simulink library "Word_Multiplexers_Lib"  (Simulink 8.7)
settings: Solver=ode45  StartTime=0.0  StopTime=10.0  RelTol=1e-3
(part 2 of 3)

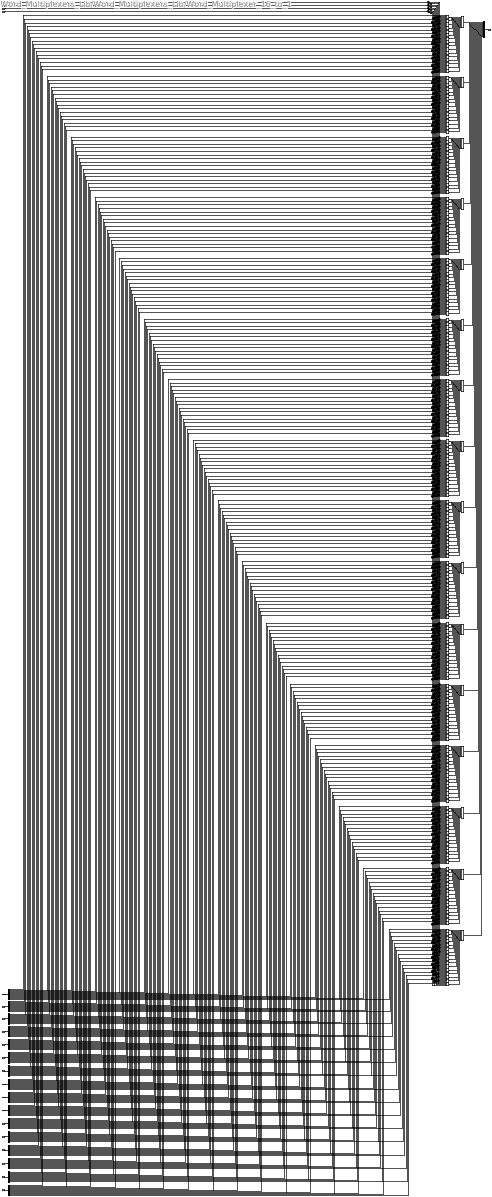
== system Word_Multiplexers_Lib/Word_Multiplexers_Lib/Word_Multiplexer_16_to_1 ==
  note: Bit_Multiplexer_16_to_1(Bit_15)
  note: Bit_Multiplexer_16_to_1(Bit_14)
  note: Bit_Multiplexer_16_to_1(Bit_13)
  note: Bit_Multiplexer_16_to_1(Bit_12)
  note: Bit_Multiplexer_16_to_1(Bit_11)
  note: Bit_Multiplexer_16_to_1(Bit_10)
  note: Bit_Multiplexer_16_to_1(Bit_09)
  note: Bit_Multiplexer_16_to_1(Bit_08)
  note: Bit_Multiplexer_16_to_1(Bit_07)
  note: Bit_Multiplexer_16_to_1(Bit_06)
  note: Bit_Multiplexer_16_to_1(Bit_05)
  note: Bit_Multiplexer_16_to_1(Bit_04)
  note: Bit_Multiplexer_16_to_1(Bit_03)
  note: Bit_Multiplexer_16_to_1(Bit_02)
  note: Bit_Multiplexer_16_to_1(Bit_01)
  note: Bit_Multiplexer_16_to_1(Bit_00)
  Address_3(1b) : Inport
  Address_2(1b) : Inport  Port=2
  Address_1(1b) : Inport  Port=3
  Address_0(1b) : Inport  Port=4
  Data_In_15(2B) : Inport  Port=5
  Data_In_14(2B) : Inport  Port=6
  Data_In_13(2B) : Inport  Port=7
  Data_In_12(2B) : Inport  Port=8
  Data_In_11(2B) : Inport  Port=9
  Data_In_10(2B) : Inport  Port=10
  Data_In_09(2B) : Inport  Port=11
  Data_In_08(2B) : Inport  Port=12
  Data_In_07(2B) : Inport  Port=13
  Data_In_06(2B) : Inport  Port=14
  Data_In_05(2B) : Inport  Port=15
  Data_In_04(2B) : Inport  Port=16
  Data_In_03(2B) : Inport  Port=17
  Data_In_02(2B) : Inport  Port=18
  Data_In_01(2B) : Inport  Port=19
  Data_In_00(2B) : Inport  Port=20
  Bus Creator : BusCreator  Inputs=16
  Bus Selector{,1..15} (16 alike) : BusSelector  OutputSignals=signal1,signal2,signal3,signal4,signal5,signal6,signal7,signal8,signal9,signal10,signal11,signal12,signal13,signal14,signal15,signal16
  Logical Operator{,1..7,13..22,26..39,42..43,47..60,63..64,68..81,84..85,89..102,105..106,110..123,126..127,131..144,147..148,152..165,168..169,173..186,189..190,194..207,210..211,215..228,231..232,236..249,252..253,257..270,273..274,278..291,294..295,299..312,315..316,320..333} (256 alike) : Logic  Inputs=5  IconShape=distinctive  AllPortsSameDT=off  OutDataTypeStr=boolean
  Logical Operator{8,40,61,82,103,124,145,166,187,208,229,250,271,292,313,334} (16 alike) : Logic  Operator=OR  Inputs=16  IconShape=distinctive  OutDataTypeStr=boolean
  Logical Operator{317..319,335} (4 alike) : Logic  Operator=NOT  Inputs=4  IconShape=distinctive  AllPortsSameDT=off  OutDataTypeStr=boolean
  Data_Out(2B) : Outport
  wires:
  Data_In_15(2B)/1 -> Bus Selector15/1
  Logical Operator103/1 -> Bus Creator/12
  Logical Operator124/1 -> Bus Creator/11
  Logical Operator145/1 -> Bus Creator/10
  Logical Operator166/1 -> Bus Creator/9
  Logical Operator82/1 -> Bus Creator/13
  Logical Operator61/1 -> Bus Creator/14
  Logical Operator40/1 -> Bus Creator/15
  Logical Operator8/1 -> Bus Creator/16
  Data_In_14(2B)/1 -> Bus Selector14/1
  Data_In_13(2B)/1 -> Bus Selector13/1
  Data_In_12(2B)/1 -> Bus Selector12/1
  Data_In_11(2B)/1 -> Bus Selector11/1
  Data_In_10(2B)/1 -> Bus Selector10/1
  Data_In_09(2B)/1 -> Bus Selector9/1
  Data_In_08(2B)/1 -> Bus Selector8/1
  Data_In_07(2B)/1 -> Bus Selector7/1
  Data_In_06(2B)/1 -> Bus Selector6/1
  Data_In_05(2B)/1 -> Bus Selector5/1
  Data_In_04(2B)/1 -> Bus Selector4/1
  Data_In_03(2B)/1 -> Bus Selector3/1
  Data_In_02(2B)/1 -> Bus Selector2/1
  Data_In_01(2B)/1 -> Bus Selector1/1
  Data_In_00(2B)/1 -> Bus Selector/1
  Bus Creator/1 -> Data_Out(2B)/1
  Logical Operator271/1 -> Bus Creator/4
  Logical Operator292/1 -> Bus Creator/3
  Logical Operator313/1 -> Bus Creator/2
  Logical Operator334/1 -> Bus Creator/1
  Logical Operator250/1 -> Bus Creator/5
  Logical Operator229/1 -> Bus Creator/6
  Logical Operator208/1 -> Bus Creator/7
  Logical Operator187/1 -> Bus Creator/8
  Logical Operator319/1 -> Logical Operator316/5, Logical Operator329/5, Logical Operator331/5, Logical Operator333/5, Logical Operator321/5, Logical Operator323/5, Logical Operator325/5, Logical Operator1/5, Logical Operator3/5, Logical Operator5/5, Logical Operator7/5, Logical Operator14/5, Logical Operator16/5, Logical Operator18/5, Logical Operator20/5, Logical Operator34/5, Logical Operator31/5, Logical Operator29/5, Logical Operator27/5, Logical Operator39/5, Logical Operator37/5, Logical Operator35/5, Logical Operator22/5, Logical Operator55/5, Logical Operator52/5, Logical Operator50/5, Logical Operator48/5, Logical Operator60/5, Logical Operator58/5, Logical Operator56/5, Logical Operator43/5, Logical Operator76/5, Logical Operator73/5, Logical Operator71/5, Logical Operator69/5, Logical Operator81/5, Logical Operator79/5, Logical Operator77/5, Logical Operator64/5, Logical Operator97/5, Logical Operator94/5, Logical Operator92/5, Logical Operator90/5, Logical Operator102/5, Logical Operator100/5, Logical Operator98/5, Logical Operator85/5, Logical Operator118/5, Logical Operator115/5, Logical Operator113/5, Logical Operator111/5, Logical Operator123/5, Logical Operator121/5, Logical Operator119/5, Logical Operator106/5, Logical Operator139/5, Logical Operator136/5, Logical Operator134/5, Logical Operator132/5, Logical Operator144/5, Logical Operator142/5, Logical Operator140/5, Logical Operator127/5, Logical Operator160/5, Logical Operator157/5, Logical Operator155/5, Logical Operator153/5, Logical Operator165/5, Logical Operator163/5, Logical Operator161/5, Logical Operator148/5, Logical Operator181/5, Logical Operator178/5, Logical Operator176/5, Logical Operator174/5, Logical Operator186/5, Logical Operator184/5, Logical Operator182/5, Logical Operator169/5, Logical Operator202/5, Logical Operator199/5, Logical Operator197/5, Logical Operator195/5, Logical Operator207/5, Logical Operator205/5, Logical Operator203/5, Logical Operator190/5, Logical Operator223/5, Logical Operator220/5, Logical Operator218/5, Logical Operator216/5, Logical Operator228/5, Logical Operator226/5, Logical Operator224/5, Logical Operator211/5, Logical Operator244/5, Logical Operator241/5, Logical Operator239/5, Logical Operator237/5, Logical Operator249/5, Logical Operator247/5, Logical Operator245/5, Logical Operator232/5, Logical Operator265/5, Logical Operator262/5, Logical Operator260/5, Logical Operator258/5, Logical Operator270/5, Logical Operator268/5, Logical Operator266/5, Logical Operator253/5, Logical Operator286/5, Logical Operator283/5, Logical Operator281/5, Logical Operator279/5, Logical Operator291/5, Logical Operator289/5, Logical Operator287/5, Logical Operator274/5, Logical Operator307/5, Logical Operator304/5, Logical Operator302/5, Logical Operator300/5, Logical Operator312/5, Logical Operator310/5, Logical Operator308/5, Logical Operator295/5, Logical Operator328/5
  Logical Operator318/1 -> Logical Operator327/4, Logical Operator329/4, Logical Operator332/4, Logical Operator333/4, Logical Operator322/4, Logical Operator323/4, Logical Operator326/4, Logical Operator34/4, Logical Operator2/4, Logical Operator3/4, Logical Operator6/4, Logical Operator7/4, Logical Operator15/4, Logical Operator16/4, Logical Operator19/4, Logical Operator20/4, Logical Operator32/4, Logical Operator29/4, Logical Operator28/4, Logical Operator39/4, Logical Operator38/4, Logical Operator35/4, Logical Operator33/4, Logical Operator55/4, Logical Operator53/4, Logical Operator50/4, Logical Operator49/4, Logical Operator60/4, Logical Operator59/4, Logical Operator56/4, Logical Operator54/4, Logical Operator76/4, Logical Operator74/4, Logical Operator71/4, Logical Operator70/4, Logical Operator81/4, Logical Operator80/4, Logical Operator77/4, Logical Operator75/4, Logical Operator97/4, Logical Operator95/4, Logical Operator92/4, Logical Operator91/4, Logical Operator102/4, Logical Operator101/4, Logical Operator98/4, Logical Operator96/4, Logical Operator118/4, Logical Operator116/4, Logical Operator113/4, Logical Operator112/4, Logical Operator123/4, Logical Operator122/4, Logical Operator119/4, Logical Operator117/4, Logical Operator139/4, Logical Operator137/4, Logical Operator134/4, Logical Operator133/4, Logical Operator144/4, Logical Operator143/4, Logical Operator140/4, Logical Operator138/4, Logical Operator160/4, Logical Operator158/4, Logical Operator155/4, Logical Operator154/4, Logical Operator165/4, Logical Operator164/4, Logical Operator161/4, Logical Operator159/4, Logical Operator181/4, Logical Operator179/4, Logical Operator176/4, Logical Operator175/4, Logical Operator186/4, Logical Operator185/4, Logical Operator182/4, Logical Operator180/4, Logical Operator202/4, Logical Operator200/4, Logical Operator197/4, Logical Operator196/4, Logical Operator207/4, Logical Operator206/4, Logical Operator203/4, Logical Operator201/4, Logical Operator223/4, Logical Operator221/4, Logical Operator218/4, Logical Operator217/4, Logical Operator228/4, Logical Operator227/4, Logical Operator224/4, Logical Operator222/4, Logical Operator244/4, Logical Operator242/4, Logical Operator239/4, Logical Operator238/4, Logical Operator249/4, Logical Operator248/4, Logical Operator245/4, Logical Operator243/4, Logical Operator265/4, Logical Operator263/4, Logical Operator260/4, Logical Operator259/4, Logical Operator270/4, Logical Operator269/4, Logical Operator266/4, Logical Operator264/4, Logical Operator286/4, Logical Operator284/4, Logical Operator281/4, Logical Operator280/4, Logical Operator291/4, Logical Operator290/4, Logical Operator287/4, Logical Operator285/4, Logical Operator307/4, Logical Operator305/4, Logical Operator302/4, Logical Operator301/4, Logical Operator312/4, Logical Operator311/4, Logical Operator308/4, Logical Operator306/4, Logical Operator328/4
  Logical Operator317/1 -> Logical Operator330/3, Logical Operator331/3, Logical Operator332/3, Logical Operator333/3, Logical Operator324/3, Logical Operator325/3, Logical Operator326/3, Logical Operator34/3, Logical Operator4/3, Logical Operator5/3, Logical Operator6/3, Logical Operator7/3, Logical Operator17/3, Logical Operator18/3, Logical Operator19/3, Logical Operator20/3, Logical Operator32/3, Logical Operator31/3, Logical Operator30/3, Logical Operator39/3, Logical Operator38/3, Logical Operator37/3, Logical Operator36/3, Logical Operator55/3, Logical Operator53/3, Logical Operator52/3, Logical Operator51/3, Logical Operator60/3, Logical Operator59/3, Logical Operator58/3, Logical Operator57/3, Logical Operator76/3, Logical Operator74/3, Logical Operator73/3, Logical Operator72/3, Logical Operator81/3, Logical Operator80/3, Logical Operator79/3, Logical Operator78/3, Logical Operator97/3, Logical Operator95/3, Logical Operator94/3, Logical Operator93/3, Logical Operator102/3, Logical Operator101/3, Logical Operator100/3, Logical Operator99/3, Logical Operator118/3, Logical Operator116/3, Logical Operator115/3, Logical Operator114/3, Logical Operator123/3, Logical Operator122/3, Logical Operator121/3, Logical Operator120/3, Logical Operator139/3, Logical Operator137/3, Logical Operator136/3, Logical Operator135/3, Logical Operator144/3, Logical Operator143/3, Logical Operator142/3, Logical Operator141/3, Logical Operator160/3, Logical Operator158/3, Logical Operator157/3, Logical Operator156/3, Logical Operator165/3, Logical Operator164/3, Logical Operator163/3, Logical Operator162/3, Logical Operator181/3, Logical Operator179/3, Logical Operator178/3, Logical Operator177/3, Logical Operator186/3, Logical Operator185/3, Logical Operator184/3, Logical Operator183/3, Logical Operator202/3, Logical Operator200/3, Logical Operator199/3, Logical Operator198/3, Logical Operator207/3, Logical Operator206/3, Logical Operator205/3, Logical Operator204/3, Logical Operator223/3, Logical Operator221/3, Logical Operator220/3, Logical Operator219/3, Logical Operator228/3, Logical Operator227/3, Logical Operator226/3, Logical Operator225/3, Logical Operator244/3, Logical Operator242/3, Logical Operator241/3, Logical Operator240/3, Logical Operator249/3, Logical Operator248/3, Logical Operator247/3, Logical Operator246/3, Logical Operator265/3, Logical Operator263/3, Logical Operator262/3, Logical Operator261/3, Logical Operator270/3, Logical Operator269/3, Logical Operator268/3, Logical Operator267/3, Logical Operator286/3, Logical Operator284/3, Logical Operator283/3, Logical Operator282/3, Logical Operator291/3, Logical Operator290/3, Logical Operator289/3, Logical Operator288/3, Logical Operator307/3, Logical Operator305/3, Logical Operator304/3, Logical Operator303/3, Logical Operator312/3, Logical Operator311/3, Logical Operator310/3, Logical Operator309/3, Logical Operator328/3
  Logical Operator335/1 -> Logical Operator320/2, Logical Operator321/2, Logical Operator322/2, Logical Operator323/2, Logical Operator324/2, Logical Operator325/2, Logical Operator326/2, Logical Operator34/2, Logical Operator13/2, Logical Operator14/2, Logical Operator15/2, Logical Operator16/2, Logical Operator17/2, Logical Operator18/2, Logical Operator19/2, Logical Operator20/2, Logical Operator32/2, Logical Operator31/2, Logical Operator30/2, Logical Operator29/2, Logical Operator28/2, Logical Operator27/2, Logical Operator26/2, Logical Operator55/2, Logical Operator53/2, Logical Operator52/2, Logical Operator51/2, Logical Operator50/2, Logical Operator49/2, Logical Operator48/2, Logical Operator47/2, Logical Operator76/2, Logical Operator74/2, Logical Operator73/2, Logical Operator72/2, Logical Operator71/2, Logical Operator70/2, Logical Operator69/2, Logical Operator68/2, Logical Operator97/2, Logical Operator95/2, Logical Operator94/2, Logical Operator93/2, Logical Operator92/2, Logical Operator91/2, Logical Operator90/2, Logical Operator89/2, Logical Operator118/2, Logical Operator116/2, Logical Operator115/2, Logical Operator114/2, Logical Operator113/2, Logical Operator112/2, Logical Operator111/2, Logical Operator110/2, Logical Operator139/2, Logical Operator137/2, Logical Operator136/2, Logical Operator135/2, Logical Operator134/2, Logical Operator133/2, Logical Operator132/2, Logical Operator131/2, Logical Operator160/2, Logical Operator158/2, Logical Operator157/2, Logical Operator156/2, Logical Operator155/2, Logical Operator154/2, Logical Operator153/2, Logical Operator152/2, Logical Operator181/2, Logical Operator179/2, Logical Operator178/2, Logical Operator177/2, Logical Operator176/2, Logical Operator175/2, Logical Operator174/2, Logical Operator173/2, Logical Operator202/2, Logical Operator200/2, Logical Operator199/2, Logical Operator198/2, Logical Operator197/2, Logical Operator196/2, Logical Operator195/2, Logical Operator194/2, Logical Operator223/2, Logical Operator221/2, Logical Operator220/2, Logical Operator219/2, Logical Operator218/2, Logical Operator217/2, Logical Operator216/2, Logical Operator215/2, Logical Operator244/2, Logical Operator242/2, Logical Operator241/2, Logical Operator240/2, Logical Operator239/2, Logical Operator238/2, Logical Operator237/2, Logical Operator236/2, Logical Operator265/2, Logical Operator263/2, Logical Operator262/2, Logical Operator261/2, Logical Operator260/2, Logical Operator259/2, Logical Operator258/2, Logical Operator257/2, Logical Operator286/2, Logical Operator284/2, Logical Operator283/2, Logical Operator282/2, Logical Operator281/2, Logical Operator280/2, Logical Operator279/2, Logical Operator278/2, Logical Operator307/2, Logical Operator305/2, Logical Operator304/2, Logical Operator303/2, Logical Operator302/2, Logical Operator301/2, Logical Operator300/2, Logical Operator299/2, Logical Operator328/2
  Bus Selector/16 -> Logical Operator20/1  "<signal16>"
  Bus Selector1/16 -> Logical Operator19/1  "<signal16>"
  Bus Selector2/16 -> Logical Operator18/1  "<signal16>"
  Bus Selector3/16 -> Logical Operator17/1  "<signal16>"
  Bus Selector4/16 -> Logical Operator16/1  "<signal16>"
  Bus Selector5/16 -> Logical Operator15/1  "<signal16>"
  Bus Selector6/16 -> Logical Operator14/1  "<signal16>"
  Bus Selector7/16 -> Logical Operator13/1  "<signal16>"
  Logical Operator20/1 -> Logical Operator8/16
  Logical Operator19/1 -> Logical Operator8/15
  Logical Operator18/1 -> Logical Operator8/14
  Logical Operator17/1 -> Logical Operator8/13
  Logical Operator16/1 -> Logical Operator8/12
  Logical Operator15/1 -> Logical Operator8/11
  Logical Operator14/1 -> Logical Operator8/10
  Logical Operator13/1 -> Logical Operator8/9
  Bus Selector15/16 -> Logical Operator/1  "<signal16>"
  Bus Selector14/16 -> Logical Operator1/1  "<signal16>"
  Bus Selector13/16 -> Logical Operator2/1  "<signal16>"
  Bus Selector12/16 -> Logical Operator3/1  "<signal16>"
  Bus Selector11/16 -> Logical Operator4/1  "<signal16>"
  Bus Selector10/16 -> Logical Operator5/1  "<signal16>"
  Bus Selector9/16 -> Logical Operator6/1  "<signal16>"
  Bus Selector8/16 -> Logical Operator7/1  "<signal16>"
  Logical Operator7/1 -> Logical Operator8/8
  Logical Operator6/1 -> Logical Operator8/7
  Logical Operator5/1 -> Logical Operator8/6
  Logical Operator4/1 -> Logical Operator8/5
  Logical Operator3/1 -> Logical Operator8/4
  Logical Operator2/1 -> Logical Operator8/3
  Logical Operator1/1 -> Logical Operator8/2
  Logical Operator/1 -> Logical Operator8/1
  Bus Selector/15 -> Logical Operator34/1  "<signal15>"
  Bus Selector1/15 -> Logical Operator32/1  "<signal15>"
  Bus Selector2/15 -> Logical Operator31/1  "<signal15>"
  Bus Selector3/15 -> Logical Operator30/1  "<signal15>"
  Bus Selector4/15 -> Logical Operator29/1  "<signal15>"
  Bus Selector5/15 -> Logical Operator28/1  "<signal15>"
  Bus Selector6/15 -> Logical Operator27/1  "<signal15>"
  Bus Selector7/15 -> Logical Operator26/1  "<signal15>"
  Logical Operator34/1 -> Logical Operator40/16
  Logical Operator32/1 -> Logical Operator40/15
  Logical Operator31/1 -> Logical Operator40/14
  Logical Operator30/1 -> Logical Operator40/13
  Logical Operator29/1 -> Logical Operator40/12
  Logical Operator28/1 -> Logical Operator40/11
  Logical Operator27/1 -> Logical Operator40/10
  Logical Operator26/1 -> Logical Operator40/9
  Bus Selector15/15 -> Logical Operator21/1  "<signal15>"
  Bus Selector14/15 -> Logical Operator22/1  "<signal15>"
  Bus Selector13/15 -> Logical Operator33/1  "<signal15>"
  Bus Selector12/15 -> Logical Operator35/1  "<signal15>"
  Bus Selector11/15 -> Logical Operator36/1  "<signal15>"
  Bus Selector10/15 -> Logical Operator37/1  "<signal15>"
  Bus Selector9/15 -> Logical Operator38/1  "<signal15>"
  Bus Selector8/15 -> Logical Operator39/1  "<signal15>"
  Logical Operator39/1 -> Logical Operator40/8
  Logical Operator38/1 -> Logical Operator40/7
  Logical Operator37/1 -> Logical Operator40/6
  Logical Operator36/1 -> Logical Operator40/5
  Logical Operator35/1 -> Logical Operator40/4
  Logical Operator33/1 -> Logical Operator40/3
  Logical Operator22/1 -> Logical Operator40/2
  Logical Operator21/1 -> Logical Operator40/1
  Bus Selector/14 -> Logical Operator55/1  "<signal14>"
  Bus Selector1/14 -> Logical Operator53/1  "<signal14>"
  Bus Selector2/14 -> Logical Operator52/1  "<signal14>"
  Bus Selector3/14 -> Logical Operator51/1  "<signal14>"
  Bus Selector4/14 -> Logical Operator50/1  "<signal14>"
  Bus Selector5/14 -> Logical Operator49/1  "<signal14>"
  Bus Selector6/14 -> Logical Operator48/1  "<signal14>"
  Bus Selector7/14 -> Logical Operator47/1  "<signal14>"
  Logical Operator55/1 -> Logical Operator61/16
  Logical Operator53/1 -> Logical Operator61/15
  Logical Operator52/1 -> Logical Operator61/14
  Logical Operator51/1 -> Logical Operator61/13
  Logical Operator50/1 -> Logical Operator61/12
  Logical Operator49/1 -> Logical Operator61/11
  Logical Operator48/1 -> Logical Operator61/10
  Logical Operator47/1 -> Logical Operator61/9
  Bus Selector15/14 -> Logical Operator42/1  "<signal14>"
  Bus Selector14/14 -> Logical Operator43/1  "<signal14>"
  Bus Selector13/14 -> Logical Operator54/1  "<signal14>"
  Bus Selector12/14 -> Logical Operator56/1  "<signal14>"
  Bus Selector11/14 -> Logical Operator57/1  "<signal14>"
  Bus Selector10/14 -> Logical Operator58/1  "<signal14>"
  Bus Selector9/14 -> Logical Operator59/1  "<signal14>"
  Bus Selector8/14 -> Logical Operator60/1  "<signal14>"
  Logical Operator60/1 -> Logical Operator61/8
  Logical Operator59/1 -> Logical Operator61/7
  Logical Operator58/1 -> Logical Operator61/6
  Logical Operator57/1 -> Logical Operator61/5
  Logical Operator56/1 -> Logical Operator61/4
  Logical Operator54/1 -> Logical Operator61/3
  Logical Operator43/1 -> Logical Operator61/2
  Logical Operator42/1 -> Logical Operator61/1
  Bus Selector/13 -> Logical Operator76/1  "<signal13>"
  Bus Selector1/13 -> Logical Operator74/1  "<signal13>"
  Bus Selector2/13 -> Logical Operator73/1  "<signal13>"
  Bus Selector3/13 -> Logical Operator72/1  "<signal13>"
  Bus Selector4/13 -> Logical Operator71/1  "<signal13>"
  Bus Selector5/13 -> Logical Operator70/1  "<signal13>"
  Bus Selector6/13 -> Logical Operator69/1  "<signal13>"
  Bus Selector7/13 -> Logical Operator68/1  "<signal13>"
  Logical Operator76/1 -> Logical Operator82/16
  Logical Operator74/1 -> Logical Operator82/15
  Logical Operator73/1 -> Logical Operator82/14
  Logical Operator72/1 -> Logical Operator82/13
  Logical Operator71/1 -> Logical Operator82/12
  Logical Operator70/1 -> Logical Operator82/11
  Logical Operator69/1 -> Logical Operator82/10
  Logical Operator68/1 -> Logical Operator82/9
  Bus Selector15/13 -> Logical Operator63/1  "<signal13>"
  Bus Selector14/13 -> Logical Operator64/1  "<signal13>"
  Bus Selector13/13 -> Logical Operator75/1  "<signal13>"
  Bus Selector12/13 -> Logical Operator77/1  "<signal13>"
  Bus Selector11/13 -> Logical Operator78/1  "<signal13>"
  Bus Selector10/13 -> Logical Operator79/1  "<signal13>"
  Bus Selector9/13 -> Logical Operator80/1  "<signal13>"
  Bus Selector8/13 -> Logical Operator81/1  "<signal13>"
  Logical Operator81/1 -> Logical Operator82/8
  Logical Operator80/1 -> Logical Operator82/7
  Logical Operator79/1 -> Logical Operator82/6
  Logical Operator78/1 -> Logical Operator82/5
  Logical Operator77/1 -> Logical Operator82/4
  Logical Operator75/1 -> Logical Operator82/3
  Logical Operator64/1 -> Logical Operator82/2
  Logical Operator63/1 -> Logical Operator82/1
  Bus Selector/12 -> Logical Operator97/1  "<signal12>"
  Bus Selector1/12 -> Logical Operator95/1  "<signal12>"
  Bus Selector2/12 -> Logical Operator94/1  "<signal12>"
  Bus Selector3/12 -> Logical Operator93/1  "<signal12>"
  Bus Selector4/12 -> Logical Operator92/1  "<signal12>"
  Bus Selector5/12 -> Logical Operator91/1  "<signal12>"
  Bus Selector6/12 -> Logical Operator90/1  "<signal12>"
  Bus Selector7/12 -> Logical Operator89/1  "<signal12>"
  Logical Operator97/1 -> Logical Operator103/16
  Logical Operator95/1 -> Logical Operator103/15
  Logical Operator94/1 -> Logical Operator103/14
  Logical Operator93/1 -> Logical Operator103/13
  Logical Operator92/1 -> Logical Operator103/12
  Logical Operator91/1 -> Logical Operator103/11
  Logical Operator90/1 -> Logical Operator103/10
  Logical Operator89/1 -> Logical Operator103/9
  Bus Selector15/12 -> Logical Operator84/1  "<signal12>"
  Bus Selector14/12 -> Logical Operator85/1  "<signal12>"
  Bus Selector13/12 -> Logical Operator96/1  "<signal12>"
  Bus Selector12/12 -> Logical Operator98/1  "<signal12>"
  Bus Selector11/12 -> Logical Operator99/1  "<signal12>"
  Bus Selector10/12 -> Logical Operator100/1  "<signal12>"
  Bus Selector9/12 -> Logical Operator101/1  "<signal12>"
  Bus Selector8/12 -> Logical Operator102/1  "<signal12>"
  Logical Operator102/1 -> Logical Operator103/8
  Logical Operator101/1 -> Logical Operator103/7
  Logical Operator100/1 -> Logical Operator103/6
  Logical Operator99/1 -> Logical Operator103/5
  Logical Operator98/1 -> Logical Operator103/4
  Logical Operator96/1 -> Logical Operator103/3
  Logical Operator85/1 -> Logical Operator103/2
  Logical Operator84/1 -> Logical Operator103/1
  Bus Selector/11 -> Logical Operator118/1  "<signal11>"
  Bus Selector1/11 -> Logical Operator116/1  "<signal11>"
  Bus Selector2/11 -> Logical Operator115/1  "<signal11>"
  Bus Selector3/11 -> Logical Operator114/1  "<signal11>"
  Bus Selector4/11 -> Logical Operator113/1  "<signal11>"
  Bus Selector5/11 -> Logical Operator112/1  "<signal11>"
  Bus Selector6/11 -> Logical Operator111/1  "<signal11>"
  Bus Selector7/11 -> Logical Operator110/1  "<signal11>"
  Logical Operator118/1 -> Logical Operator124/16
  Logical Operator116/1 -> Logical Operator124/15
  Logical Operator115/1 -> Logical Operator124/14
  Logical Operator114/1 -> Logical Operator124/13
  Logical Operator113/1 -> Logical Operator124/12
  Logical Operator112/1 -> Logical Operator124/11
  Logical Operator111/1 -> Logical Operator124/10
  Logical Operator110/1 -> Logical Operator124/9
  Bus Selector15/11 -> Logical Operator105/1  "<signal11>"
  Bus Selector14/11 -> Logical Operator106/1  "<signal11>"
  Bus Selector13/11 -> Logical Operator117/1  "<signal11>"
  Bus Selector12/11 -> Logical Operator119/1  "<signal11>"
  Bus Selector11/11 -> Logical Operator120/1  "<signal11>"
  Bus Selector10/11 -> Logical Operator121/1  "<signal11>"
  Bus Selector9/11 -> Logical Operator122/1  "<signal11>"
  Bus Selector8/11 -> Logical Operator123/1  "<signal11>"
  Logical Operator123/1 -> Logical Operator124/8
  Logical Operator122/1 -> Logical Operator124/7
  Logical Operator121/1 -> Logical Operator124/6
  Logical Operator120/1 -> Logical Operator124/5
  Logical Operator119/1 -> Logical Operator124/4
  Logical Operator117/1 -> Logical Operator124/3
  Logical Operator106/1 -> Logical Operator124/2
  Logical Operator105/1 -> Logical Operator124/1
  Bus Selector/10 -> Logical Operator139/1  "<signal10>"
  Bus Selector1/10 -> Logical Operator137/1  "<signal10>"
  Bus Selector2/10 -> Logical Operator136/1  "<signal10>"
  Bus Selector3/10 -> Logical Operator135/1  "<signal10>"
  Bus Selector4/10 -> Logical Operator134/1  "<signal10>"
  Bus Selector5/10 -> Logical Operator133/1  "<signal10>"
  Bus Selector6/10 -> Logical Operator132/1  "<signal10>"
  Bus Selector7/10 -> Logical Operator131/1  "<signal10>"
  Logical Operator139/1 -> Logical Operator145/16
  Logical Operator137/1 -> Logical Operator145/15
  Logical Operator136/1 -> Logical Operator145/14
  Logical Operator135/1 -> Logical Operator145/13
  Logical Operator134/1 -> Logical Operator145/12
  Logical Operator133/1 -> Logical Operator145/11
  Logical Operator132/1 -> Logical Operator145/10
  Logical Operator131/1 -> Logical Operator145/9
  Bus Selector15/10 -> Logical Operator126/1  "<signal10>"
  Bus Selector14/10 -> Logical Operator127/1  "<signal10>"
  Bus Selector13/10 -> Logical Operator138/1  "<signal10>"
  Bus Selector12/10 -> Logical Operator140/1  "<signal10>"
  Bus Selector11/10 -> Logical Operator141/1  "<signal10>"
  Bus Selector10/10 -> Logical Operator142/1  "<signal10>"
  Bus Selector9/10 -> Logical Operator143/1  "<signal10>"
  Bus Selector8/10 -> Logical Operator144/1  "<signal10>"
  Logical Operator144/1 -> Logical Operator145/8
  Logical Operator143/1 -> Logical Operator145/7
  Logical Operator142/1 -> Logical Operator145/6
  Logical Operator141/1 -> Logical Operator145/5
  Logical Operator140/1 -> Logical Operator145/4
  Logical Operator138/1 -> Logical Operator145/3
  Logical Operator127/1 -> Logical Operator145/2
  Logical Operator126/1 -> Logical Operator145/1
  Bus Selector/9 -> Logical Operator160/1  "<signal9>"
  Bus Selector1/9 -> Logical Operator158/1  "<signal9>"
  Bus Selector2/9 -> Logical Operator157/1  "<signal9>"
  Bus Selector3/9 -> Logical Operator156/1  "<signal9>"
  Bus Selector4/9 -> Logical Operator155/1  "<signal9>"
  Bus Selector5/9 -> Logical Operator154/1  "<signal9>"
  Bus Selector6/9 -> Logical Operator153/1  "<signal9>"
  Bus Selector7/9 -> Logical Operator152/1  "<signal9>"
  Logical Operator160/1 -> Logical Operator166/16
  Logical Operator158/1 -> Logical Operator166/15
  Logical Operator157/1 -> Logical Operator166/14
  Logical Operator156/1 -> Logical Operator166/13
  Logical Operator155/1 -> Logical Operator166/12
  Logical Operator154/1 -> Logical Operator166/11
  Logical Operator153/1 -> Logical Operator166/10
  Logical Operator152/1 -> Logical Operator166/9
  Bus Selector15/9 -> Logical Operator147/1  "<signal9>"
  Bus Selector14/9 -> Logical Operator148/1  "<signal9>"
  Bus Selector13/9 -> Logical Operator159/1  "<signal9>"
  Bus Selector12/9 -> Logical Operator161/1  "<signal9>"
  Bus Selector11/9 -> Logical Operator162/1  "<signal9>"
  Bus Selector10/9 -> Logical Operator163/1  "<signal9>"
  Bus Selector9/9 -> Logical Operator164/1  "<signal9>"
  Bus Selector8/9 -> Logical Operator165/1  "<signal9>"
  Logical Operator165/1 -> Logical Operator166/8
  Logical Operator164/1 -> Logical Operator166/7
  Logical Operator163/1 -> Logical Operator166/6
  Logical Operator162/1 -> Logical Operator166/5
  Logical Operator161/1 -> Logical Operator166/4
  Logical Operator159/1 -> Logical Operator166/3
  Logical Operator148/1 -> Logical Operator166/2
  Logical Operator147/1 -> Logical Operator166/1
  Bus Selector/8 -> Logical Operator181/1  "<signal8>"
  Bus Selector1/8 -> Logical Operator179/1  "<signal8>"
  Bus Selector2/8 -> Logical Operator178/1  "<signal8>"
  Bus Selector3/8 -> Logical Operator177/1  "<signal8>"
  Bus Selector4/8 -> Logical Operator176/1  "<signal8>"
  Bus Selector5/8 -> Logical Operator175/1  "<signal8>"
  Bus Selector6/8 -> Logical Operator174/1  "<signal8>"
  Bus Selector7/8 -> Logical Operator173/1  "<signal8>"
  Logical Operator181/1 -> Logical Operator187/16
  Logical Operator179/1 -> Logical Operator187/15
  Logical Operator178/1 -> Logical Operator187/14
  Logical Operator177/1 -> Logical Operator187/13
  Logical Operator176/1 -> Logical Operator187/12
  Logical Operator175/1 -> Logical Operator187/11
  Logical Operator174/1 -> Logical Operator187/10
  Logical Operator173/1 -> Logical Operator187/9
  Bus Selector15/8 -> Logical Operator168/1  "<signal8>"
  Bus Selector14/8 -> Logical Operator169/1  "<signal8>"
  Bus Selector13/8 -> Logical Operator180/1  "<signal8>"
  Bus Selector12/8 -> Logical Operator182/1  "<signal8>"
  Bus Selector11/8 -> Logical Operator183/1  "<signal8>"
  Bus Selector10/8 -> Logical Operator184/1  "<signal8>"
  Bus Selector9/8 -> Logical Operator185/1  "<signal8>"
  Bus Selector8/8 -> Logical Operator186/1  "<signal8>"
  Logical Operator186/1 -> Logical Operator187/8
  Logical Operator185/1 -> Logical Operator187/7
  Logical Operator184/1 -> Logical Operator187/6
  Logical Operator183/1 -> Logical Operator187/5
  Logical Operator182/1 -> Logical Operator187/4
  Logical Operator180/1 -> Logical Operator187/3
  Logical Operator169/1 -> Logical Operator187/2
  Logical Operator168/1 -> Logical Operator187/1
  Bus Selector/7 -> Logical Operator202/1  "<signal7>"
  Bus Selector1/7 -> Logical Operator200/1  "<signal7>"
  Bus Selector2/7 -> Logical Operator199/1  "<signal7>"
  Bus Selector3/7 -> Logical Operator198/1  "<signal7>"
  Bus Selector4/7 -> Logical Operator197/1  "<signal7>"
  Bus Selector5/7 -> Logical Operator196/1  "<signal7>"
  Bus Selector6/7 -> Logical Operator195/1  "<signal7>"
  Bus Selector7/7 -> Logical Operator194/1  "<signal7>"
  Logical Operator202/1 -> Logical Operator208/16
  Logical Operator200/1 -> Logical Operator208/15
  Logical Operator199/1 -> Logical Operator208/14
  Logical Operator198/1 -> Logical Operator208/13
  Logical Operator197/1 -> Logical Operator208/12
  Logical Operator196/1 -> Logical Operator208/11
  Logical Operator195/1 -> Logical Operator208/10
  Logical Operator194/1 -> Logical Operator208/9
  Bus Selector15/7 -> Logical Operator189/1  "<signal7>"
  Bus Selector14/7 -> Logical Operator190/1  "<signal7>"
  Bus Selector13/7 -> Logical Operator201/1  "<signal7>"
  Bus Selector12/7 -> Logical Operator203/1  "<signal7>"
  Bus Selector11/7 -> Logical Operator204/1  "<signal7>"
  Bus Selector10/7 -> Logical Operator205/1  "<signal7>"
  Bus Selector9/7 -> Logical Operator206/1  "<signal7>"
  Bus Selector8/7 -> Logical Operator207/1  "<signal7>"
  Logical Operator207/1 -> Logical Operator208/8
  Logical Operator206/1 -> Logical Operator208/7
  Logical Operator205/1 -> Logical Operator208/6
  Logical Operator204/1 -> Logical Operator208/5
  Logical Operator203/1 -> Logical Operator208/4
  Logical Operator201/1 -> Logical Operator208/3
  Logical Operator190/1 -> Logical Operator208/2
  Logical Operator189/1 -> Logical Operator208/1
  Bus Selector/6 -> Logical Operator223/1  "<signal6>"
  Bus Selector1/6 -> Logical Operator221/1  "<signal6>"
  Bus Selector2/6 -> Logical Operator220/1  "<signal6>"
  Bus Selector3/6 -> Logical Operator219/1  "<signal6>"
  Bus Selector4/6 -> Logical Operator218/1  "<signal6>"
  Bus Selector5/6 -> Logical Operator217/1  "<signal6>"
  Bus Selector6/6 -> Logical Operator216/1  "<signal6>"
  Bus Selector7/6 -> Logical Operator215/1  "<signal6>"
  Logical Operator223/1 -> Logical Operator229/16
  Logical Operator221/1 -> Logical Operator229/15
  Logical Operator220/1 -> Logical Operator229/14
  Logical Operator219/1 -> Logical Operator229/13
  Logical Operator218/1 -> Logical Operator229/12
  Logical Operator217/1 -> Logical Operator229/11
  Logical Operator216/1 -> Logical Operator229/10
  Logical Operator215/1 -> Logical Operator229/9
  Bus Selector15/6 -> Logical Operator210/1  "<signal6>"
  Bus Selector14/6 -> Logical Operator211/1  "<signal6>"
  Bus Selector13/6 -> Logical Operator222/1  "<signal6>"
  Bus Selector12/6 -> Logical Operator224/1  "<signal6>"
  Bus Selector11/6 -> Logical Operator225/1  "<signal6>"
  Bus Selector10/6 -> Logical Operator226/1  "<signal6>"
  Bus Selector9/6 -> Logical Operator227/1  "<signal6>"
  Bus Selector8/6 -> Logical Operator228/1  "<signal6>"
  Logical Operator228/1 -> Logical Operator229/8
  Logical Operator227/1 -> Logical Operator229/7
  Logical Operator226/1 -> Logical Operator229/6
  Logical Operator225/1 -> Logical Operator229/5
  Logical Operator224/1 -> Logical Operator229/4
  Logical Operator222/1 -> Logical Operator229/3
  Logical Operator211/1 -> Logical Operator229/2
  Logical Operator210/1 -> Logical Operator229/1
  Bus Selector/5 -> Logical Operator244/1  "<signal5>"
  Bus Selector1/5 -> Logical Operator242/1  "<signal5>"
  Bus Selector2/5 -> Logical Operator241/1  "<signal5>"
  Bus Selector3/5 -> Logical Operator240/1  "<signal5>"
  Bus Selector4/5 -> Logical Operator239/1  "<signal5>"
  Bus Selector5/5 -> Logical Operator238/1  "<signal5>"
  Bus Selector6/5 -> Logical Operator237/1  "<signal5>"
  Bus Selector7/5 -> Logical Operator236/1  "<signal5>"
  Logical Operator244/1 -> Logical Operator250/16
  Logical Operator242/1 -> Logical Operator250/15
  Logical Operator241/1 -> Logical Operator250/14
  Logical Operator240/1 -> Logical Operator250/13
  Logical Operator239/1 -> Logical Operator250/12
  Logical Operator238/1 -> Logical Operator250/11
  Logical Operator237/1 -> Logical Operator250/10
  Logical Operator236/1 -> Logical Operator250/9
  Bus Selector15/5 -> Logical Operator231/1  "<signal5>"
  Bus Selector14/5 -> Logical Operator232/1  "<signal5>"
  Bus Selector13/5 -> Logical Operator243/1  "<signal5>"
  Bus Selector12/5 -> Logical Operator245/1  "<signal5>"
  Bus Selector11/5 -> Logical Operator246/1  "<signal5>"
  Bus Selector10/5 -> Logical Operator247/1  "<signal5>"
  Bus Selector9/5 -> Logical Operator248/1  "<signal5>"
  Bus Selector8/5 -> Logical Operator249/1  "<signal5>"
  Logical Operator249/1 -> Logical Operator250/8
  Logical Operator248/1 -> Logical Operator250/7
  Logical Operator247/1 -> Logical Operator250/6
  Logical Operator246/1 -> Logical Operator250/5
  Logical Operator245/1 -> Logical Operator250/4
  Logical Operator243/1 -> Logical Operator250/3
  Logical Operator232/1 -> Logical Operator250/2
  Logical Operator231/1 -> Logical Operator250/1
  Bus Selector/4 -> Logical Operator265/1  "<signal4>"
  Bus Selector1/4 -> Logical Operator263/1  "<signal4>"
  Bus Selector2/4 -> Logical Operator262/1  "<signal4>"
  Bus Selector3/4 -> Logical Operator261/1  "<signal4>"
  Bus Selector4/4 -> Logical Operator260/1  "<signal4>"
  Bus Selector5/4 -> Logical Operator259/1  "<signal4>"
  Bus Selector6/4 -> Logical Operator258/1  "<signal4>"
  Bus Selector7/4 -> Logical Operator257/1  "<signal4>"
  Logical Operator265/1 -> Logical Operator271/16
  Logical Operator263/1 -> Logical Operator271/15
  Logical Operator262/1 -> Logical Operator271/14
  Logical Operator261/1 -> Logical Operator271/13
  Logical Operator260/1 -> Logical Operator271/12
  Logical Operator259/1 -> Logical Operator271/11
  Logical Operator258/1 -> Logical Operator271/10
  Logical Operator257/1 -> Logical Operator271/9
  Bus Selector15/4 -> Logical Operator252/1  "<signal4>"
  Bus Selector14/4 -> Logical Operator253/1  "<signal4>"
  Bus Selector13/4 -> Logical Operator264/1  "<signal4>"
  Bus Selector12/4 -> Logical Operator266/1  "<signal4>"
  Bus Selector11/4 -> Logical Operator267/1  "<signal4>"
  Bus Selector10/4 -> Logical Operator268/1  "<signal4>"
  Bus Selector9/4 -> Logical Operator269/1  "<signal4>"
  Bus Selector8/4 -> Logical Operator270/1  "<signal4>"
  Logical Operator270/1 -> Logical Operator271/8
  Logical Operator269/1 -> Logical Operator271/7
  Logical Operator268/1 -> Logical Operator271/6
  Logical Operator267/1 -> Logical Operator271/5
  Logical Operator266/1 -> Logical Operator271/4
  Logical Operator264/1 -> Logical Operator271/3
  Logical Operator253/1 -> Logical Operator271/2
  Logical Operator252/1 -> Logical Operator271/1
  Bus Selector/3 -> Logical Operator286/1  "<signal3>"
  Bus Selector1/3 -> Logical Operator284/1  "<signal3>"
  Bus Selector2/3 -> Logical Operator283/1  "<signal3>"
  Bus Selector3/3 -> Logical Operator282/1  "<signal3>"
  Bus Selector4/3 -> Logical Operator281/1  "<signal3>"
  Bus Selector5/3 -> Logical Operator280/1  "<signal3>"
  Bus Selector6/3 -> Logical Operator279/1  "<signal3>"
  Bus Selector7/3 -> Logical Operator278/1  "<signal3>"
  Logical Operator286/1 -> Logical Operator292/16
  Logical Operator284/1 -> Logical Operator292/15
  Logical Operator283/1 -> Logical Operator292/14
  Logical Operator282/1 -> Logical Operator292/13
  Logical Operator281/1 -> Logical Operator292/12
  Logical Operator280/1 -> Logical Operator292/11
  Logical Operator279/1 -> Logical Operator292/10
  Logical Operator278/1 -> Logical Operator292/9
  Bus Selector15/3 -> Logical Operator273/1  "<signal3>"
  Bus Selector14/3 -> Logical Operator274/1  "<signal3>"
  Bus Selector13/3 -> Logical Operator285/1  "<signal3>"
  Bus Selector12/3 -> Logical Operator287/1  "<signal3>"
  Bus Selector11/3 -> Logical Operator288/1  "<signal3>"
  Bus Selector10/3 -> Logical Operator289/1  "<signal3>"
  Bus Selector9/3 -> Logical Operator290/1  "<signal3>"
  Bus Selector8/3 -> Logical Operator291/1  "<signal3>"
  Logical Operator291/1 -> Logical Operator292/8
  Logical Operator290/1 -> Logical Operator292/7
  Logical Operator289/1 -> Logical Operator292/6
  Logical Operator288/1 -> Logical Operator292/5
  Logical Operator287/1 -> Logical Operator292/4
  Logical Operator285/1 -> Logical Operator292/3
  Logical Operator274/1 -> Logical Operator292/2
  Logical Operator273/1 -> Logical Operator292/1
  Bus Selector/2 -> Logical Operator307/1  "<signal2>"
  Bus Selector1/2 -> Logical Operator305/1  "<signal2>"
  Bus Selector2/2 -> Logical Operator304/1  "<signal2>"
  Bus Selector3/2 -> Logical Operator303/1  "<signal2>"
  Bus Selector4/2 -> Logical Operator302/1  "<signal2>"
  Bus Selector5/2 -> Logical Operator301/1  "<signal2>"
  Bus Selector6/2 -> Logical Operator300/1  "<signal2>"
  Bus Selector7/2 -> Logical Operator299/1  "<signal2>"
  Logical Operator307/1 -> Logical Operator313/16
  Logical Operator305/1 -> Logical Operator313/15
  Logical Operator304/1 -> Logical Operator313/14
  Logical Operator303/1 -> Logical Operator313/13
  Logical Operator302/1 -> Logical Operator313/12
  Logical Operator301/1 -> Logical Operator313/11
  Logical Operator300/1 -> Logical Operator313/10
  Logical Operator299/1 -> Logical Operator313/9
  Bus Selector15/2 -> Logical Operator294/1  "<signal2>"
  Bus Selector14/2 -> Logical Operator295/1  "<signal2>"
  Bus Selector13/2 -> Logical Operator306/1  "<signal2>"
  Bus Selector12/2 -> Logical Operator308/1  "<signal2>"
  Bus Selector11/2 -> Logical Operator309/1  "<signal2>"
  Bus Selector10/2 -> Logical Operator310/1  "<signal2>"
  Bus Selector9/2 -> Logical Operator311/1  "<signal2>"
  Bus Selector8/2 -> Logical Operator312/1  "<signal2>"
  Logical Operator312/1 -> Logical Operator313/8
  Logical Operator311/1 -> Logical Operator313/7
  Logical Operator310/1 -> Logical Operator313/6
  Logical Operator309/1 -> Logical Operator313/5
  Logical Operator308/1 -> Logical Operator313/4
  Logical Operator306/1 -> Logical Operator313/3
  Logical Operator295/1 -> Logical Operator313/2
  Logical Operator294/1 -> Logical Operator313/1
  Address_0(1b)/1 -> Logical Operator319/1, Logical Operator/5, Logical Operator2/5, Logical Operator4/5, Logical Operator6/5, Logical Operator13/5, Logical Operator15/5, Logical Operator17/5, Logical Operator19/5, Logical Operator32/5, Logical Operator30/5, Logical Operator28/5, Logical Operator26/5, Logical Operator38/5, Logical Operator36/5, Logical Operator33/5, Logical Operator21/5, Logical Operator53/5, Logical Operator51/5, Logical Operator49/5, Logical Operator47/5, Logical Operator59/5, Logical Operator57/5, Logical Operator54/5, Logical Operator42/5, Logical Operator74/5, Logical Operator72/5, Logical Operator70/5, Logical Operator68/5, Logical Operator80/5, Logical Operator78/5, Logical Operator75/5, Logical Operator63/5, Logical Operator95/5, Logical Operator93/5, Logical Operator91/5, Logical Operator89/5, Logical Operator101/5, Logical Operator99/5, Logical Operator96/5, Logical Operator84/5, Logical Operator116/5, Logical Operator114/5, Logical Operator112/5, Logical Operator110/5, Logical Operator122/5, Logical Operator120/5, Logical Operator117/5, Logical Operator105/5, Logical Operator137/5, Logical Operator135/5, Logical Operator133/5, Logical Operator131/5, Logical Operator143/5, Logical Operator141/5, Logical Operator138/5, Logical Operator126/5, Logical Operator158/5, Logical Operator156/5, Logical Operator154/5, Logical Operator152/5, Logical Operator164/5, Logical Operator162/5, Logical Operator159/5, Logical Operator147/5, Logical Operator179/5, Logical Operator177/5, Logical Operator175/5, Logical Operator173/5, Logical Operator185/5, Logical Operator183/5, Logical Operator180/5, Logical Operator168/5, Logical Operator200/5, Logical Operator198/5, Logical Operator196/5, Logical Operator194/5, Logical Operator206/5, Logical Operator204/5, Logical Operator201/5, Logical Operator189/5, Logical Operator221/5, Logical Operator219/5, Logical Operator217/5, Logical Operator215/5, Logical Operator227/5, Logical Operator225/5, Logical Operator222/5, Logical Operator210/5, Logical Operator242/5, Logical Operator240/5, Logical Operator238/5, Logical Operator236/5, Logical Operator248/5, Logical Operator246/5, Logical Operator243/5, Logical Operator231/5, Logical Operator263/5, Logical Operator261/5, Logical Operator259/5, Logical Operator257/5, Logical Operator269/5, Logical Operator267/5, Logical Operator264/5, Logical Operator252/5, Logical Operator284/5, Logical Operator282/5, Logical Operator280/5, Logical Operator278/5, Logical Operator290/5, Logical Operator288/5, Logical Operator285/5, Logical Operator273/5, Logical Operator305/5, Logical Operator303/5, Logical Operator301/5, Logical Operator299/5, Logical Operator311/5, Logical Operator309/5, Logical Operator306/5, Logical Operator294/5, Logical Operator326/5, Logical Operator324/5, Logical Operator322/5, Logical Operator320/5, Logical Operator332/5, Logical Operator330/5, Logical Operator327/5, Logical Operator315/5
  Address_1(1b)/1 -> Logical Operator318/1, Logical Operator/4, Logical Operator1/4, Logical Operator4/4, Logical Operator5/4, Logical Operator13/4, Logical Operator14/4, Logical Operator17/4, Logical Operator18/4, Logical Operator31/4, Logical Operator30/4, Logical Operator27/4, Logical Operator26/4, Logical Operator37/4, Logical Operator36/4, Logical Operator22/4, Logical Operator21/4, Logical Operator52/4, Logical Operator51/4, Logical Operator48/4, Logical Operator47/4, Logical Operator58/4, Logical Operator57/4, Logical Operator43/4, Logical Operator42/4, Logical Operator73/4, Logical Operator72/4, Logical Operator69/4, Logical Operator68/4, Logical Operator79/4, Logical Operator78/4, Logical Operator64/4, Logical Operator63/4, Logical Operator94/4, Logical Operator93/4, Logical Operator90/4, Logical Operator89/4, Logical Operator100/4, Logical Operator99/4, Logical Operator85/4, Logical Operator84/4, Logical Operator115/4, Logical Operator114/4, Logical Operator111/4, Logical Operator110/4, Logical Operator121/4, Logical Operator120/4, Logical Operator106/4, Logical Operator105/4, Logical Operator136/4, Logical Operator135/4, Logical Operator132/4, Logical Operator131/4, Logical Operator142/4, Logical Operator141/4, Logical Operator127/4, Logical Operator126/4, Logical Operator157/4, Logical Operator156/4, Logical Operator153/4, Logical Operator152/4, Logical Operator163/4, Logical Operator162/4, Logical Operator148/4, Logical Operator147/4, Logical Operator178/4, Logical Operator177/4, Logical Operator174/4, Logical Operator173/4, Logical Operator184/4, Logical Operator183/4, Logical Operator169/4, Logical Operator168/4, Logical Operator199/4, Logical Operator198/4, Logical Operator195/4, Logical Operator194/4, Logical Operator205/4, Logical Operator204/4, Logical Operator190/4, Logical Operator189/4, Logical Operator220/4, Logical Operator219/4, Logical Operator216/4, Logical Operator215/4, Logical Operator226/4, Logical Operator225/4, Logical Operator211/4, Logical Operator210/4, Logical Operator241/4, Logical Operator240/4, Logical Operator237/4, Logical Operator236/4, Logical Operator247/4, Logical Operator246/4, Logical Operator232/4, Logical Operator231/4, Logical Operator262/4, Logical Operator261/4, Logical Operator258/4, Logical Operator257/4, Logical Operator268/4, Logical Operator267/4, Logical Operator253/4, Logical Operator252/4, Logical Operator283/4, Logical Operator282/4, Logical Operator279/4, Logical Operator278/4, Logical Operator289/4, Logical Operator288/4, Logical Operator274/4, Logical Operator273/4, Logical Operator304/4, Logical Operator303/4, Logical Operator300/4, Logical Operator299/4, Logical Operator310/4, Logical Operator309/4, Logical Operator295/4, Logical Operator294/4, Logical Operator325/4, Logical Operator324/4, Logical Operator321/4, Logical Operator320/4, Logical Operator331/4, Logical Operator330/4, Logical Operator316/4, Logical Operator315/4
  Address_2(1b)/1 -> Logical Operator317/1, Logical Operator/3, Logical Operator1/3, Logical Operator2/3, Logical Operator3/3, Logical Operator13/3, Logical Operator14/3, Logical Operator15/3, Logical Operator16/3, Logical Operator29/3, Logical Operator28/3, Logical Operator27/3, Logical Operator26/3, Logical Operator35/3, Logical Operator33/3, Logical Operator22/3, Logical Operator21/3, Logical Operator50/3, Logical Operator49/3, Logical Operator48/3, Logical Operator47/3, Logical Operator56/3, Logical Operator54/3, Logical Operator43/3, Logical Operator42/3, Logical Operator71/3, Logical Operator70/3, Logical Operator69/3, Logical Operator68/3, Logical Operator77/3, Logical Operator75/3, Logical Operator64/3, Logical Operator63/3, Logical Operator92/3, Logical Operator91/3, Logical Operator90/3, Logical Operator89/3, Logical Operator98/3, Logical Operator96/3, Logical Operator85/3, Logical Operator84/3, Logical Operator113/3, Logical Operator112/3, Logical Operator111/3, Logical Operator110/3, Logical Operator119/3, Logical Operator117/3, Logical Operator106/3, Logical Operator105/3, Logical Operator134/3, Logical Operator133/3, Logical Operator132/3, Logical Operator131/3, Logical Operator140/3, Logical Operator138/3, Logical Operator127/3, Logical Operator126/3, Logical Operator155/3, Logical Operator154/3, Logical Operator153/3, Logical Operator152/3, Logical Operator161/3, Logical Operator159/3, Logical Operator148/3, Logical Operator147/3, Logical Operator176/3, Logical Operator175/3, Logical Operator174/3, Logical Operator173/3, Logical Operator182/3, Logical Operator180/3, Logical Operator169/3, Logical Operator168/3, Logical Operator197/3, Logical Operator196/3, Logical Operator195/3, Logical Operator194/3, Logical Operator203/3, Logical Operator201/3, Logical Operator190/3, Logical Operator189/3, Logical Operator218/3, Logical Operator217/3, Logical Operator216/3, Logical Operator215/3, Logical Operator224/3, Logical Operator222/3, Logical Operator211/3, Logical Operator210/3, Logical Operator239/3, Logical Operator238/3, Logical Operator237/3, Logical Operator236/3, Logical Operator245/3, Logical Operator243/3, Logical Operator232/3, Logical Operator231/3, Logical Operator260/3, Logical Operator259/3, Logical Operator258/3, Logical Operator257/3, Logical Operator266/3, Logical Operator264/3, Logical Operator253/3, Logical Operator252/3, Logical Operator281/3, Logical Operator280/3, Logical Operator279/3, Logical Operator278/3, Logical Operator287/3, Logical Operator285/3, Logical Operator274/3, Logical Operator273/3, Logical Operator302/3, Logical Operator301/3, Logical Operator300/3, Logical Operator299/3, Logical Operator308/3, Logical Operator306/3, Logical Operator295/3, Logical Operator294/3, Logical Operator323/3, Logical Operator322/3, Logical Operator321/3, Logical Operator320/3, Logical Operator329/3, Logical Operator327/3, Logical Operator316/3, Logical Operator315/3
  Address_3(1b)/1 -> Logical Operator335/1, Logical Operator/2, Logical Operator1/2, Logical Operator2/2, Logical Operator3/2, Logical Operator4/2, Logical Operator5/2, Logical Operator6/2, Logical Operator7/2, Logical Operator39/2, Logical Operator38/2, Logical Operator37/2, Logical Operator36/2, Logical Operator35/2, Logical Operator33/2, Logical Operator22/2, Logical Operator21/2, Logical Operator60/2, Logical Operator59/2, Logical Operator58/2, Logical Operator57/2, Logical Operator56/2, Logical Operator54/2, Logical Operator43/2, Logical Operator42/2, Logical Operator81/2, Logical Operator80/2, Logical Operator79/2, Logical Operator78/2, Logical Operator77/2, Logical Operator75/2, Logical Operator64/2, Logical Operator63/2, Logical Operator102/2, Logical Operator101/2, Logical Operator100/2, Logical Operator99/2, Logical Operator98/2, Logical Operator96/2, Logical Operator85/2, Logical Operator84/2, Logical Operator123/2, Logical Operator122/2, Logical Operator121/2, Logical Operator120/2, Logical Operator119/2, Logical Operator117/2, Logical Operator106/2, Logical Operator105/2, Logical Operator144/2, Logical Operator143/2, Logical Operator142/2, Logical Operator141/2, Logical Operator140/2, Logical Operator138/2, Logical Operator127/2, Logical Operator126/2, Logical Operator165/2, Logical Operator164/2, Logical Operator163/2, Logical Operator162/2, Logical Operator161/2, Logical Operator159/2, Logical Operator148/2, Logical Operator147/2, Logical Operator186/2, Logical Operator185/2, Logical Operator184/2, Logical Operator183/2, Logical Operator182/2, Logical Operator180/2, Logical Operator169/2, Logical Operator168/2, Logical Operator207/2, Logical Operator206/2, Logical Operator205/2, Logical Operator204/2, Logical Operator203/2, Logical Operator201/2, Logical Operator190/2, Logical Operator189/2, Logical Operator228/2, Logical Operator227/2, Logical Operator226/2, Logical Operator225/2, Logical Operator224/2, Logical Operator222/2, Logical Operator211/2, Logical Operator210/2, Logical Operator249/2, Logical Operator248/2, Logical Operator247/2, Logical Operator246/2, Logical Operator245/2, Logical Operator243/2, Logical Operator232/2, Logical Operator231/2, Logical Operator270/2, Logical Operator269/2, Logical Operator268/2, Logical Operator267/2, Logical Operator266/2, Logical Operator264/2, Logical Operator253/2, Logical Operator252/2, Logical Operator291/2, Logical Operator290/2, Logical Operator289/2, Logical Operator288/2, Logical Operator287/2, Logical Operator285/2, Logical Operator274/2, Logical Operator273/2, Logical Operator312/2, Logical Operator311/2, Logical Operator310/2, Logical Operator309/2, Logical Operator308/2, Logical Operator306/2, Logical Operator295/2, Logical Operator294/2, Logical Operator333/2, Logical Operator332/2, Logical Operator331/2, Logical Operator330/2, Logical Operator329/2, Logical Operator327/2, Logical Operator316/2, Logical Operator315/2
  Bus Selector/1 -> Logical Operator328/1  "<signal1>"
  Bus Selector1/1 -> Logical Operator326/1  "<signal1>"
  Bus Selector2/1 -> Logical Operator325/1  "<signal1>"
  Bus Selector3/1 -> Logical Operator324/1  "<signal1>"
  Bus Selector4/1 -> Logical Operator323/1  "<signal1>"
  Bus Selector5/1 -> Logical Operator322/1  "<signal1>"
  Bus Selector6/1 -> Logical Operator321/1  "<signal1>"
  Bus Selector7/1 -> Logical Operator320/1  "<signal1>"
  Logical Operator328/1 -> Logical Operator334/16
  Logical Operator326/1 -> Logical Operator334/15
  Logical Operator325/1 -> Logical Operator334/14
  Logical Operator324/1 -> Logical Operator334/13
  Logical Operator323/1 -> Logical Operator334/12
  Logical Operator322/1 -> Logical Operator334/11
  Logical Operator321/1 -> Logical Operator334/10
  Logical Operator320/1 -> Logical Operator334/9
  Bus Selector15/1 -> Logical Operator315/1  "<signal1>"
  Bus Selector14/1 -> Logical Operator316/1  "<signal1>"
  Bus Selector13/1 -> Logical Operator327/1  "<signal1>"
  Bus Selector12/1 -> Logical Operator329/1  "<signal1>"
  Bus Selector11/1 -> Logical Operator330/1  "<signal1>"
  Bus Selector10/1 -> Logical Operator331/1  "<signal1>"
  Bus Selector9/1 -> Logical Operator332/1  "<signal1>"
  Bus Selector8/1 -> Logical Operator333/1  "<signal1>"
  Logical Operator333/1 -> Logical Operator334/8
  Logical Operator332/1 -> Logical Operator334/7
  Logical Operator331/1 -> Logical Operator334/6
  Logical Operator330/1 -> Logical Operator334/5
  Logical Operator329/1 -> Logical Operator334/4
  Logical Operator327/1 -> Logical Operator334/3
  Logical Operator316/1 -> Logical Operator334/2
  Logical Operator315/1 -> Logical Operator334/1
